simulink model "coarse_fine_tracking_system"  (R2023a)
settings: Solver=VariableStepAuto  StartTime=0.0  StopTime=50  FixedStep=0.1  RelTol=1e-3
values from neighbouring files (symbols this model uses):
  Dm = zeros(2,2)    [setup.m]
  Dp = diag([1 1])    [setup.m]
  epsilon = [0; 0]    [setup.m]
  f_a_sup = [10; 10]    [setup.m]
  INITIAL_LOWER_OBSERVER_VALUE = -INITIAL_UPPER_OBSERVER_VALUE    [setup.m]
  INITIAL_SYSTEM_VALUE = [0.3946 0.4599 -0.7478 -0.3090 -0.9610 0.0815]'    [setup.m]
  INITIAL_UPPER_OBSERVER_VALUE = [1 1 30 1 1 30]'    [setup.m]
  K = blkdiag(A_1,A_2)    [setup.m]
  L = [L_1 L_2; L_3 L_4]    [setup.m]
  M_E = blkdiag(M_1r,M_2r)    [setup.m]
  P = blkdiag(P_1,P_2)    [setup.m]
  Phi_E = blkdiag(Phi_A_1,Phi_A_2)    [setup.m]
  varepsilon_l = -varepsilon_u    [setup.m]
  varepsilon_u = [0.1 0.1 0.1 0.1 0.1 0.1]'    [setup.m]
  w_l = -w_u    [setup.m]
  w_u = [1; 1]    [setup.m]
settings Model: Creator=weijie  LastModifiedBy=weijie
settings DataIOCC: ReturnWorkspaceOutputs=off

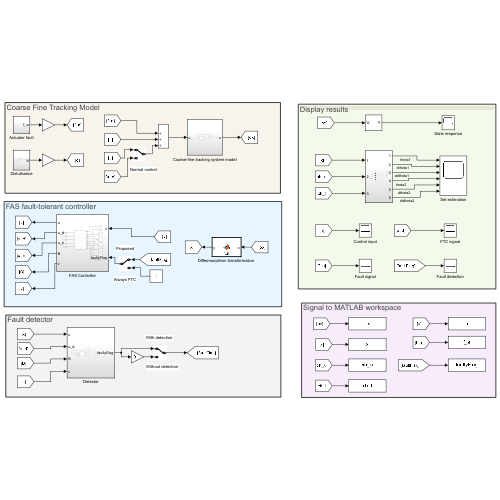
[thumbnail: Simulink's stored preview of the top-level diagram]
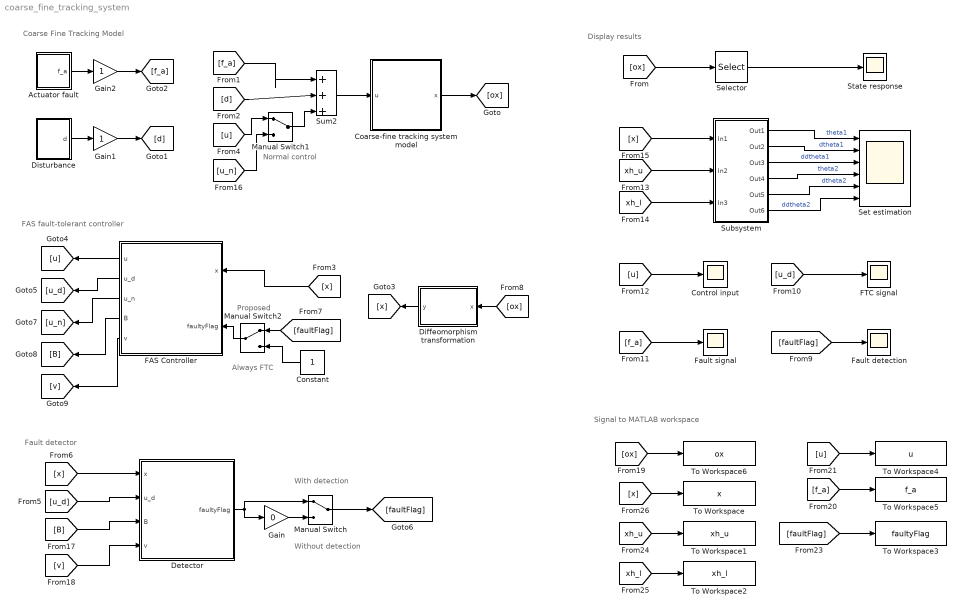
== system coarse_fine_tracking_system ==
  note: Proposed
  note: Signal to MATLAB workspace
  note: Display results
  note: FAS fault-tolerant controller
  note: Fault detector
  note: Coarse Fine Tracking Model
  note: Always FTC
  note: Normal control
  note: Without detection
  note: With detection
  Actuator fault : Subsystem
  Coarse-fine tracking system model : Subsystem
  Constant : Constant
  Control input : Scope
  Detector : Subsystem
  "Diffeomorphism transformation " : MATLAB Function  TreatAsAtomicUnit=on
  Disturbance : Subsystem
  FAS Controller : Subsystem
  FTC signal : Scope
  Fault detection : Scope
  Fault signal : Scope
  Gain : Gain  Gain=0
  Gain1 : Gain
  Gain2 : Gain
  Manual Switch : ManualSwitch
  Manual Switch1 : ManualSwitch
  Manual Switch2 : ManualSwitch
  Selector : Selector  InputPortWidth=6  IndexOptions=Index vector (dialog)  Indices=[1 2 4 5]  OutputSizes=1
  Set estimation : Scope  NumInputPorts=6
  State response : Scope
  Subsystem : Subsystem
  Sum2 : Sum  Inputs=|+++
  To Workspace : ToWorkspace  VariableName=x  SaveFormat=Structure With Time  SampleTime=-1
  To Workspace1 : ToWorkspace  VariableName=xh_u  SaveFormat=Structure With Time  SampleTime=-1
  To Workspace2 : ToWorkspace  VariableName=xh_l  SaveFormat=Structure With Time  SampleTime=-1
  To Workspace3 : ToWorkspace  VariableName=faultyFlag  SaveFormat=Structure With Time  SampleTime=-1
  To Workspace4 : ToWorkspace  VariableName=u  SaveFormat=Structure With Time  SampleTime=-1
  To Workspace5 : ToWorkspace  VariableName=f_a  SaveFormat=Structure With Time  SampleTime=-1
  To Workspace6 : ToWorkspace  VariableName=ox  SaveFormat=Structure With Time  SampleTime=-1
  wires:
  Sum2/1 -> Coarse-fine tracking system model/1(u)
  [f_a] -> Sum2/1
  Selector/1 -> State response/1
  [ox] -> Selector/1
  [x] -> FAS Controller/1(x)
  [d] -> Sum2/2
  Coarse-fine tracking system model/1(x) -> [ox]
  Actuator fault/1(f_a) -> Gain2/1
  Disturbance/1(d) -> Gain1/1
  "Diffeomorphism transformation "/1(y) -> [x]
  FAS Controller/1(u) -> [u]
  [u] -> Manual Switch1/1
  FAS Controller/2(u_d) -> [u_d]
  [u_d] -> Detector/2(u_d)
  [x] -> Detector/1(x)
  Detector/1(faultyFlag) -> Manual Switch/1, Gain/1
  [faultFlag] -> Manual Switch2/1
  [ox] -> "Diffeomorphism transformation "/1(x)
  [faultFlag] -> Fault detection/1
  [u_d] -> FTC signal/1
  [f_a] -> Fault signal/1
  [u] -> Control input/1
  FAS Controller/3(u_n) -> [u_n]
  Manual Switch/1 -> [faultFlag]
  Gain/1 -> Manual Switch/2
  Manual Switch1/1 -> Sum2/3
  [u_n] -> Manual Switch1/2
  Manual Switch2/1 -> FAS Controller/2(faultyFlag)
  Constant/1 -> Manual Switch2/2
  Gain1/1 -> [d]
  Gain2/1 -> [f_a]
  FAS Controller/4(B) -> [B]
  [B] -> Detector/3(B)
  FAS Controller/5(v) -> [v]
  [v] -> Detector/4(v)
  [x] -> Subsystem/1(In1)
  [xh_u] -> Subsystem/2(In2)
  [xh_l] -> Subsystem/3(In3)
  Subsystem/1(Out1) -> Set estimation/1  "theta1"
  Subsystem/2(Out2) -> Set estimation/2  "dtheta1"
  Subsystem/3(Out3) -> Set estimation/3  "ddtheta1"
  Subsystem/4(Out4) -> Set estimation/4  "theta2"
  Subsystem/5(Out5) -> Set estimation/5  "dtheta2"
  Subsystem/6(Out6) -> Set estimation/6  "ddtheta2"
  [f_a] -> To Workspace5/1
  [u] -> To Workspace4/1
  [ox] -> To Workspace6/1
  [xh_u] -> To Workspace1/1
  [xh_l] -> To Workspace2/1
  [x] -> To Workspace/1
  [faultFlag] -> To Workspace3/1

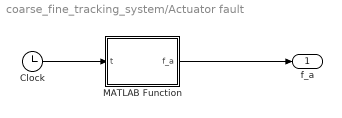
== system coarse_fine_tracking_system/Actuator fault ==
  Clock : Clock
  MATLAB Function : MATLAB Function  TreatAsAtomicUnit=on
  f_a : Outport
  wires:
  Clock/1 -> MATLAB Function/1(t)
  MATLAB Function/1(f_a) -> f_a/1

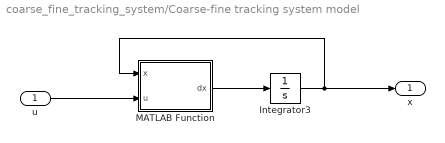
== system coarse_fine_tracking_system/Coarse-fine tracking system model ==
  u : Inport
  Integrator3 : Integrator  InitialCondition=INITIAL_SYSTEM_VALUE
  MATLAB Function : MATLAB Function  TreatAsAtomicUnit=on
  x : Outport
  wires:
  Integrator3/1 -> x/1, MATLAB Function/1(x)
  MATLAB Function/1(dx) -> Integrator3/1
  u/1 -> MATLAB Function/2(u)

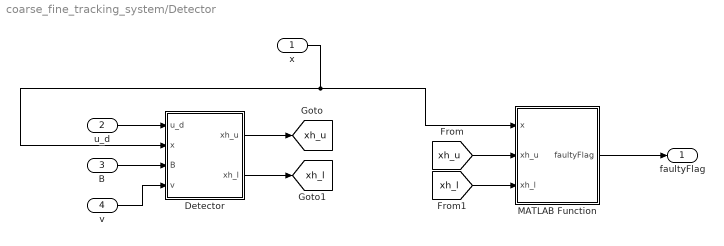
== system coarse_fine_tracking_system/Detector ==
  x : Inport
  u_d : Inport  Port=2
  B : Inport  Port=3
  v : Inport  Port=4
  Detector : Subsystem
  MATLAB Function : MATLAB Function  TreatAsAtomicUnit=on
  faultyFlag : Outport
  tag scope: xh_l=global, xh_u=global
  wires:
  Detector/1(xh_u) -> [xh_u]
  u_d/1 -> Detector/1(u_d)
  x/1 -> MATLAB Function/1(x), Detector/2(x)
  MATLAB Function/1(faultyFlag) -> faultyFlag/1
  Detector/2(xh_l) -> [xh_l]
  [xh_u] -> MATLAB Function/2(xh_u)
  [xh_l] -> MATLAB Function/3(xh_l)
  B/1 -> Detector/3(B)
  v/1 -> Detector/4(v)

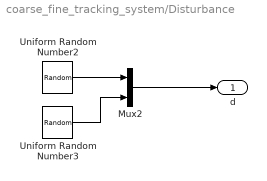
== system coarse_fine_tracking_system/Disturbance ==
  Mux2 : Mux  Inputs=2
  Uniform Random Number2 : UniformRandomNumber  Minimum=-w_u(1)  Maximum=w_u(1)  SampleTime=0.05
  Uniform Random Number3 : UniformRandomNumber  Minimum=-w_u(2)  Maximum=w_u(2)  Seed=1  SampleTime=0.05
  d : Outport
  wires:
  Uniform Random Number3/1 -> Mux2/2
  Uniform Random Number2/1 -> Mux2/1
  Mux2/1 -> d/1

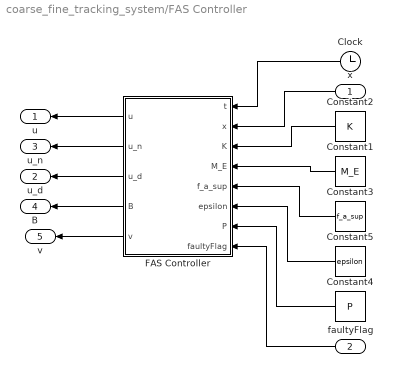
== system coarse_fine_tracking_system/FAS Controller ==
  x : Inport
  faultyFlag : Inport  Port=2
  Clock : Clock
  Constant1 : Constant  Value=M_E  VectorParams1D=off
  Constant2 : Constant  Value=K  VectorParams1D=off
  Constant3 : Constant  Value=f_a_sup  VectorParams1D=off
  Constant4 : Constant  Value=P  VectorParams1D=off
  Constant5 : Constant  Value=epsilon  VectorParams1D=off
  FAS Controller : MATLAB Function  TreatAsAtomicUnit=on
  u : Outport
  u_d : Outport  Port=2
  u_n : Outport  Port=3
  B : Outport  Port=4
  v : Outport  Port=5
  wires:
  Constant1/1 -> FAS Controller/4(M_E)
  faultyFlag/1 -> FAS Controller/8(faultyFlag)
  Constant4/1 -> FAS Controller/7(P)
  FAS Controller/1(u) -> u/1
  Constant2/1 -> FAS Controller/3(K)
  Constant3/1 -> FAS Controller/5(f_a_sup)
  x/1 -> FAS Controller/2(x)
  FAS Controller/3(u_d) -> u_d/1
  FAS Controller/2(u_n) -> u_n/1
  Constant5/1 -> FAS Controller/6(epsilon)
  FAS Controller/4(B) -> B/1
  Clock/1 -> FAS Controller/1(t)
  FAS Controller/5(v) -> v/1

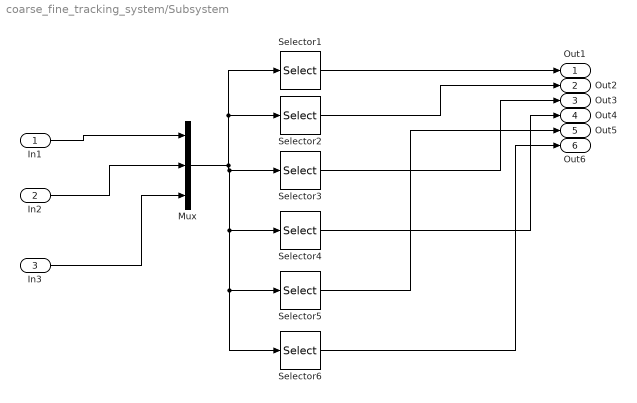
== system coarse_fine_tracking_system/Subsystem ==
  In1 : Inport
  In2 : Inport  Port=2
  In3 : Inport  Port=3
  Mux : Mux  Inputs=3
  Selector1 : Selector  InputPortWidth=18  IndexOptions=Index vector (dialog)  Indices=[1 7 13]  OutputSizes=1
  Selector2 : Selector  InputPortWidth=18  IndexOptions=Index vector (dialog)  Indices=[2 8 14]  OutputSizes=1
  Selector3 : Selector  InputPortWidth=18  IndexOptions=Index vector (dialog)  Indices=[3 9 15]  OutputSizes=1
  Selector4 : Selector  InputPortWidth=18  IndexOptions=Index vector (dialog)  Indices=[4 10 16]  OutputSizes=1
  Selector5 : Selector  InputPortWidth=18  IndexOptions=Index vector (dialog)  Indices=[5 11 17]  OutputSizes=1
  Selector6 : Selector  InputPortWidth=18  IndexOptions=Index vector (dialog)  Indices=[6 12 18]  OutputSizes=1
  Out1 : Outport
  Out2 : Outport  Port=2
  Out3 : Outport  Port=3
  Out4 : Outport  Port=4
  Out5 : Outport  Port=5
  Out6 : Outport  Port=6
  wires:
  In3/1 -> Mux/3
  In2/1 -> Mux/2
  Mux/1 -> Selector2/1, Selector1/1, Selector6/1, Selector5/1, Selector4/1, Selector3/1
  Selector5/1 -> Out5/1
  Selector4/1 -> Out4/1
  Selector2/1 -> Out2/1
  In1/1 -> Mux/1
  Selector3/1 -> Out3/1
  Selector6/1 -> Out6/1
  Selector1/1 -> Out1/1

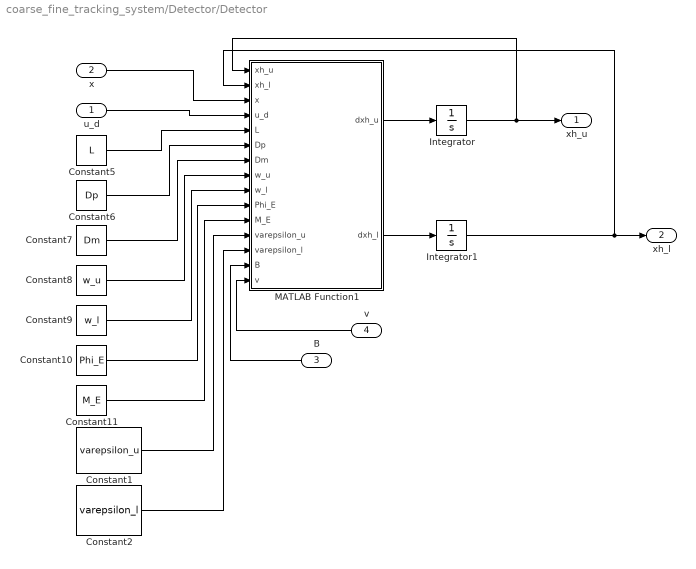
== system coarse_fine_tracking_system/Detector/Detector ==
  u_d : Inport
  x : Inport  Port=2
  B : Inport  Port=3
  v : Inport  Port=4
  Constant1 : Constant  Value=varepsilon_u  VectorParams1D=off
  Constant10 : Constant  Value=Phi_E  VectorParams1D=off
  Constant11 : Constant  Value=M_E  VectorParams1D=off
  Constant2 : Constant  Value=varepsilon_l  VectorParams1D=off
  Constant5 : Constant  Value=L  VectorParams1D=off
  Constant6 : Constant  Value=Dp  VectorParams1D=off
  Constant7 : Constant  Value=Dm  VectorParams1D=off
  Constant8 : Constant  Value=w_u  VectorParams1D=off
  Constant9 : Constant  Value=w_l  VectorParams1D=off
  Integrator : Integrator  InitialCondition=INITIAL_UPPER_OBSERVER_VALUE
  Integrator1 : Integrator  InitialCondition=INITIAL_LOWER_OBSERVER_VALUE
  MATLAB Function1 : MATLAB Function  TreatAsAtomicUnit=on
  xh_u : Outport
  xh_l : Outport  Port=2
  wires:
  MATLAB Function1/1(dxh_u) -> Integrator/1
  Constant9/1 -> MATLAB Function1/9(w_l)
  Constant10/1 -> MATLAB Function1/10(Phi_E)
  Constant8/1 -> MATLAB Function1/8(w_u)
  Constant11/1 -> MATLAB Function1/11(M_E)
  MATLAB Function1/2(dxh_l) -> Integrator1/1
  Constant5/1 -> MATLAB Function1/5(L)
  Constant7/1 -> MATLAB Function1/7(Dm)
  Constant6/1 -> MATLAB Function1/6(Dp)
  x/1 -> MATLAB Function1/3(x)
  u_d/1 -> MATLAB Function1/4(u_d)
  Integrator/1 -> MATLAB Function1/1(xh_u), xh_u/1
  Integrator1/1 -> MATLAB Function1/2(xh_l), xh_l/1
  Constant1/1 -> MATLAB Function1/12(varepsilon_u)
  Constant2/1 -> MATLAB Function1/13(varepsilon_l)
  B/1 -> MATLAB Function1/14(B)
  v/1 -> MATLAB Function1/15(v)

== matlab function coarse_fine_tracking_system/FAS Controller/FAS Controller ==
  data: t input; x input; u output; u_n output; K input; M_E input; f_a_sup input; epsilon input; u_d output; P input; faultyFlag input; B output; v output
function [u,u_n,u_d,B,v] = fcn(t,x,K,M_E,f_a_sup,epsilon,P,faultyFlag)
theta_1 = x(1);
dtheta_1 = x(2);
ddtheta_1 = x(3);
theta_2 = x(4);
dtheta_2 = x(5);
ddtheta_2 = x(6);

c_1 = 1; c_2 = 1;
a_1 = 1; a_2 = 1;
D_1 = 20*dtheta_1*sin(theta_1);
K_1 = 15*cos(theta_1);
M_2 = 2 + cos(theta_2);
D_2 = dtheta_2*sin(theta_2);
K_2 = 2*cos(theta_2);

pD1_ptheta1 = 20*dtheta_1*cos(theta_1);
pD1_pdtheta1 = 20*sin(theta_1);
pK1_ptheta1 = -15*sin(theta_1);
pM2_ptheta2 = -sin(theta_2);
pD2_ptheta2 = dtheta_2*cos(theta_2);
pD2_pdtheta2 = sin(theta_2);
pK2_ptheta2 = -2*sin(theta_2);

f_1 = -pD1_ptheta1*dtheta_1^2 - pD1_pdtheta1*dtheta_1*ddtheta_1 - D_1*ddtheta_1 ...
      -pK1_ptheta1*dtheta_1 - a_1*ddtheta_1 - a_1*D_1*dtheta_1 - a_1*K_1;
tf_2 = pM2_ptheta2*dtheta_2*ddtheta_2 + pD2_ptheta2*dtheta_2^2 ...
       +pD2_pdtheta2*dtheta_2*ddtheta_2 + D_2*ddtheta_2 + pK2_ptheta2*dtheta_2 ...
       +a_2*M_2*ddtheta_2 + a_2*D_2*dtheta_2 + a_2*K_2;
f_2 = -M_2 \ tf_2;
f = [f_1; f_2 - c_2/M_2*theta_1];
B = diag([c_1 c_2/M_2]);

v = [10; 10]*sin(t)*0;
u_ast = K*x;
u_n = -B \ (f + u_ast - v);
u_d = -sign((2*x'*P*M_E*B)').*(f_a_sup + epsilon)*faultyFlag*1;
u = u_n + u_d;

== matlab function coarse_fine_tracking_system/Coarse-fine tracking system model/MATLAB Function ==
  data: x input; u input; dx output
function dx = fcn(x,u)
u_1 = u(1);
u_2 = u(2);
theta_1 = x(1);
dtheta_1 = x(2);
tau_1 = x(3);
theta_2 = x(4);
dtheta_2 = x(5);
tau_2 = x(6);

c_1 = 1; c_2 = 1;
a_1 = 1; a_2 = 1;
D_1 = 20*dtheta_1*sin(theta_1);
K_1 = 15*cos(theta_1);
M_2 = 2 + cos(theta_2);
D_2 = dtheta_2*sin(theta_2);
K_2 = 2*cos(theta_2);

dx = [dtheta_1;
      -D_1*dtheta_1 - K_1 + tau_1;
      -a_1*tau_1 + c_1*u_1;
      dtheta_2;
      M_2 \ ( -D_2*dtheta_2 - K_2 + tau_2 );
       -c_2*theta_1 - a_2*tau_2 + c_2*u_2];

== matlab function coarse_fine_tracking_system/Diffeomorphism transformation  ==
  data: x input; y output
function y = fcn(x)
theta_1 = x(1);
dtheta_1 = x(2);
tau_1 = x(3);
theta_2 = x(4);
dtheta_2 = x(5);
tau_2 = x(6);

c_1 = 1; c_2 = 1;
a_1 = 1; a_2 = 1;
D_1 = 20*dtheta_1*sin(theta_1);
K_1 = 15*cos(theta_1);
M_2 = 2 + cos(theta_2);
D_2 = dtheta_2*sin(theta_2);
K_2 = 2*cos(theta_2);

ddtheta_1 = -D_1*dtheta_1 - K_1 + tau_1;
ddtheta_2 = M_2 \ ( -D_2*dtheta_2 - K_2 + tau_2 );

y = [theta_1;
     dtheta_1;
     ddtheta_1;
     theta_2;
     dtheta_2;
     ddtheta_2];

== matlab function coarse_fine_tracking_system/Detector/Detector/MATLAB Function1 ==
  data: xh_u input; xh_l input; x input; u_d input; L input; Dp input; Dm input; w_u input; w_l input; Phi_E input; M_E input; varepsilon_u input; varepsilon_l input; B input; v input; dxh_u output; dxh_l output
function [dxh_u, dxh_l] = fcn(xh_u,xh_l,x,u_d,L,Dp,Dm,w_u,w_l,Phi_E,M_E,varepsilon_u,varepsilon_l,B,v)
c = 0.0;
M_E1 = [c	c;
        c	c;
        1	c;
        c	c;
        c	c;
        c	1];
dxh_u = Phi_E*xh_u + L*(x - xh_u) + M_E1*Dp*w_u + M_E1*Dm*w_l + M_E*B*u_d*1 + varepsilon_u + M_E*v;
dxh_l = Phi_E*xh_l + L*(x - xh_l) + M_E1*Dp*w_l + M_E1*Dm*w_u + M_E*B*u_d*1 + varepsilon_l + M_E*v;

== matlab function coarse_fine_tracking_system/Detector/MATLAB Function ==
  data: x input; xh_u input; faultyFlag output; xh_l input
function faultyFlag = fcn(x,xh_u,xh_l)
if max(x > xh_u) || max(x < xh_l)
    faultyFlag = 1;
else
    faultyFlag = 0;
end

== matlab function coarse_fine_tracking_system/Actuator fault/MATLAB Function ==
  data: t input; f_a output
function f_a = fcn(t)
if t >= 20 && t <= 40
    f_a = [9 + 1*sin(2*t);
           6 + 0.1*t];
else
    f_a = [0; 0];
end
